simulink model "crane_izka"  (R2021a)
settings: Solver=VariableStepAuto  StartTime=0.0  StopTime=sim_time  FixedStep=sim_step  MaxStep=sim_step  RelTol=1e-3
values from neighbouring files (symbols this model uses):
  C = Pop(i,4)    [GA.m]    (also in izka.mat = 4.74862786183; meranie1.mat = 11.3345130893; meranie2.mat = 10.8395112259; meranie3.mat = 10.5647928076)
  F_cart_den = [0.09763	1	0]    [GA.m]    (also in izka.mat = [2.81374905355e-05 1 0]; meranie1.mat = [2.81374905355e-05 1 0]; meranie2.mat = [2.81374905355e-05 1 0]; meranie3.mat = [2.81374905355e-05 1 0])
  F_cart_num = [0	0	0.3345]    [GA.m]    (also in izka.mat = [0 0 0.21759813997]; meranie1.mat = [0 0 0.21759813997]; meranie2.mat = [0 0 0.21759813997]; meranie3.mat = [0 0 0.21759813997])
  F_pend_den = [1	0.01135	12.54]    [GA.m]    (also in izka.mat = [1 0.0125366535497 12.956800497]; meranie1.mat = [1 0.0125366535497 12.956800497]; meranie2.mat = [1 0.0125366535497 12.956800497]; meranie3.mat = [1 0.0125366535497 12.956800497])
  F_pend_num = [-1.214 0	0]    [GA.m]    (also in izka.mat = [-1.37069413494 0 0]; meranie1.mat = [-1.37069413494 0 0]; meranie2.mat = [-1.37069413494 0 0]; meranie3.mat = [-1.37069413494 0 0])
  I = Pop(i,2)    [GA.m]    (also in izka.mat = 7.78140484293; meranie1.mat = 0.526099986265; meranie2.mat = 3.05318784953; meranie3.mat = 0.594304323923)
  I1 = Pop(i,3)    [GA.m]    (also in meranie_6_4.mat = -16.7252340033)
  l = 0.58    [GA.m]    (also in izka.mat; meranie1.mat; meranie2.mat; meranie3.mat)
  P = Pop(i,1)    [GA.m]    (also in izka.mat = 9.77813174253; meranie1.mat = 6.16880734651; meranie2.mat = 6.25392782724; meranie3.mat = 8.1585790558)
  P1 = 6.16880734651    [meranie1.mat]    (also in meranie2.mat = 6.25392782724)
  sim_step = 0.01    [GA.m]    (also in meranie1.mat; meranie2.mat; meranie3.mat; meranie4-2.mat)
libraries: pid_lib x4, simulink x4, SignalEditorBlockLib x2
settings Model: Creator=maros-pc  LastModifiedBy=maros-pc
settings SolverCC: ConsecutiveZCsStepRelTol=10000*128*eps
settings DebuggingCC: UnconnectedInputMsg=none  UnconnectedOutputMsg=none  UnconnectedLineMsg=none
settings ModelReferenceCC: EnableRefExpFcnMdlSchedulingChecks=off
settings RTWCC: Description=Generic Real-Time Target  DLArmComputeVersion=20.02.1

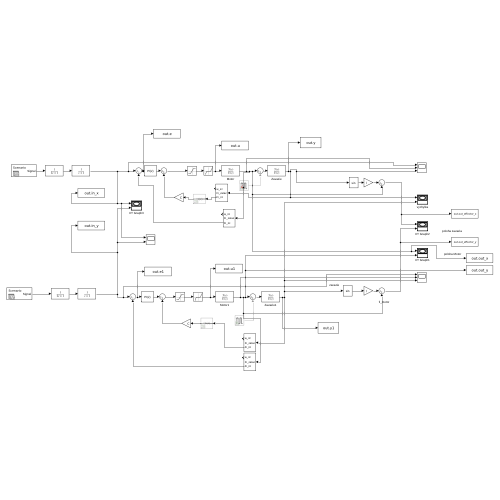
[thumbnail: Simulink's stored preview of the top-level diagram]
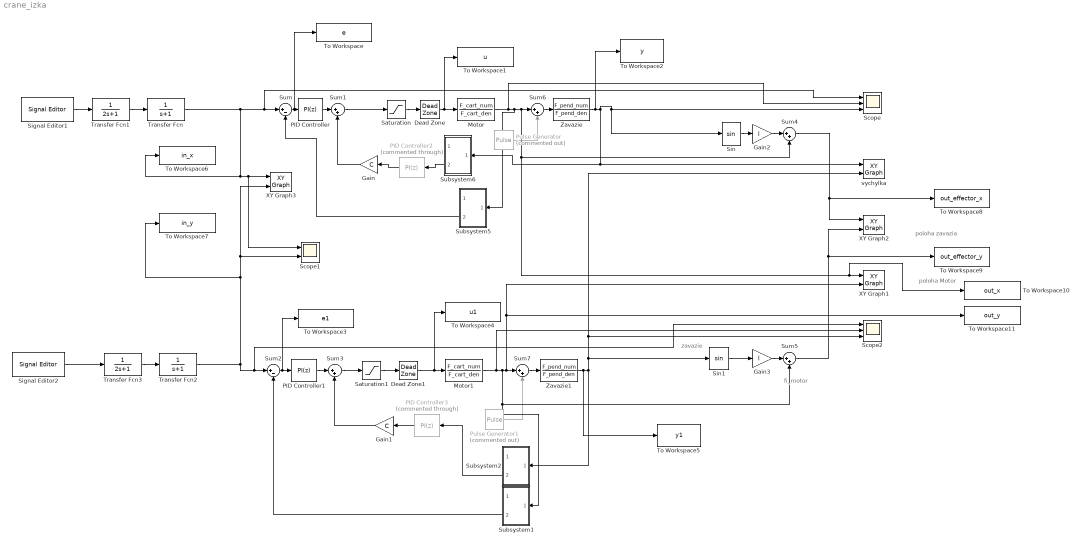
== system crane_izka ==
  note: poloha zavazia
  note: poloha Motor
  note: fi_motor
  note: zavazie
  Dead Zone : DeadZone  LowerValue=-0.2  UpperValue=0.2  SaturateOnIntegerOverflow=on
  Dead Zone1 : DeadZone  LowerValue=-0.2  UpperValue=0.2  SaturateOnIntegerOverflow=on
  Gain : Gain  Gain=C
  Gain1 : Gain  Gain=C
  Gain2 : Gain  Gain=l
  Gain3 : Gain  Gain=l
  Motor : TransferFcn  Numerator=F_cart_num  Denominator=F_cart_den
  Motor1 : TransferFcn  Numerator=F_cart_num  Denominator=F_cart_den
  PID Controller : pid_lib/PID Controller  Controller=PI  Form=Parallel  TimeDomain=Discrete-time  UseExternalTs=off  SampleTime=-1  IntegratorMethod=Forward Euler  FilterMethod=Forward Euler  ControllerParametersSource=internal  P=P  I=I  D=0  N=100  UseFilter=on  TunerSelectOption=Transfer Function Based (PID Tuner App)  InitialConditionSource=internal  InitialConditionForIntegrator=0  InitialConditionForFilter=0  DifferentiatorICPrevScaledInput=0  ExternalReset=none  TrackingMode=off  Kt=1  LimitOutput=off  SatLimitsSource=internal  UpperSaturationLimit=inf  LowerSaturationLimit=-inf  LinearizeAsGain=on  AntiWindupMode=none  Kb=1  POutMin=[]  POutMax=[]  IOutMin=[]  IOutMax=[]  DOutMin=[]  DOutMax=[]  NOutMin=[]  NOutMax=[]  SumOutMin=[]  SumOutMax=[]  SaturationOutMin=[]  SaturationOutMax=[]  PParamMin=[]  PParamMax=[]  IParamMin=[]  IParamMax=[]  DParamMin=[]  DParamMax=[]  NParamMin=[]  NParamMax=[]  KbParamMin=[]  KbParamMax=[]  KtParamMin=[]  KtParamMax=[]  KbOutMin=[]  KbOutMax=[]  KtOutMin=[]  KtOutMax=[]  IntegratorOutMin=[]  IntegratorOutMax=[]  FilterOutMin=[]  FilterOutMax=[]  SumI1OutMin=[]  SumI1OutMax=[]  SumI2OutMin=[]  SumI2OutMax=[]  SumI3OutMin=[]  SumI3OutMax=[]  SumI4OutMin=[]  SumI4OutMax=[]  SumDOutMin=[]  SumDOutMax=[]  DifferentiatorOutMin=[]  DifferentiatorOutMax=[]  FilterDiffOutCoefMin=[]  FilterDiffOutCoefMax=[]  ReciprocalOutMin=[]  ReciprocalOutMax=[]  SumDenOutMin=[]  SumDenOutMax=[]  SumNumOutMin=[]  SumNumOutMax=[]  DivideOutMin=[]  DivideOutMax=[]  UdiffTsProdOutMin=[]  UdiffTsProdOutMax=[]  NTsProdOutMin=[]  NTsProdOutMax=[]  UintegralTsProdOutMin=[]  UintegralTsProdOutMax=[]  UngainTsProdOutMin=[]  UngainTsProdOutMax=[]  IntegratorContinuousStateAttributes=''  IntegratorStateMustResolveToSignalObject=off  IntegratorRTWStateStorageClass=Auto  FilterContinuousStateAttributes=''  FilterStateMustResolveToSignalObject=off  FilterRTWStateStorageClass=Auto  ParallelPVariant=InternalParameters  IdealPVariant=Disabled  IVariant=InternalParameters  DVariant=Disabled  IntegratorVariant=Discrete  SatVariant=Disabled  AWVariant=Passthrough  PCopyVariant=Disabled  TRVariant=Disabled  FdbkBlocksVariant=Forward  IdealPFdbkVariant=Disabled  SatFdbkVariant=Disabled  DerivativeFilterVariant=Disabled  NVariant=Disabled  NCopyVariant=Disabled_SignalSpec  FilterICVariant=Disabled  IntegratorICVariant=InternalICs  ExternalResetVariant=Disabled  TRSumVariant=Passthrough  SumFdbkVariant=Disabled  SumVariant=Sum_PI  TsampFilterVariant=InternalTs  TsampNgainVariant=Passthrough  TsampIntegralVariant=Disabled_SignalSpec  ExternalSaturationOutDataTypeStr=Inherit: Same as second input
  PID Controller1 : pid_lib/PID Controller  Controller=PI  Form=Parallel  TimeDomain=Discrete-time  UseExternalTs=off  SampleTime=-1  IntegratorMethod=Forward Euler  FilterMethod=Forward Euler  ControllerParametersSource=internal  P=P  I=I  D=0  N=100  UseFilter=on  TunerSelectOption=Transfer Function Based (PID Tuner App)  InitialConditionSource=internal  InitialConditionForIntegrator=0  InitialConditionForFilter=0  DifferentiatorICPrevScaledInput=0  ExternalReset=none  TrackingMode=off  Kt=1  LimitOutput=off  SatLimitsSource=internal  UpperSaturationLimit=inf  LowerSaturationLimit=-inf  LinearizeAsGain=on  AntiWindupMode=none  Kb=1  POutMin=[]  POutMax=[]  IOutMin=[]  IOutMax=[]  DOutMin=[]  DOutMax=[]  NOutMin=[]  NOutMax=[]  SumOutMin=[]  SumOutMax=[]  SaturationOutMin=[]  SaturationOutMax=[]  PParamMin=[]  PParamMax=[]  IParamMin=[]  IParamMax=[]  DParamMin=[]  DParamMax=[]  NParamMin=[]  NParamMax=[]  KbParamMin=[]  KbParamMax=[]  KtParamMin=[]  KtParamMax=[]  KbOutMin=[]  KbOutMax=[]  KtOutMin=[]  KtOutMax=[]  IntegratorOutMin=[]  IntegratorOutMax=[]  FilterOutMin=[]  FilterOutMax=[]  SumI1OutMin=[]  SumI1OutMax=[]  SumI2OutMin=[]  SumI2OutMax=[]  SumI3OutMin=[]  SumI3OutMax=[]  SumI4OutMin=[]  SumI4OutMax=[]  SumDOutMin=[]  SumDOutMax=[]  DifferentiatorOutMin=[]  DifferentiatorOutMax=[]  FilterDiffOutCoefMin=[]  FilterDiffOutCoefMax=[]  ReciprocalOutMin=[]  ReciprocalOutMax=[]  SumDenOutMin=[]  SumDenOutMax=[]  SumNumOutMin=[]  SumNumOutMax=[]  DivideOutMin=[]  DivideOutMax=[]  UdiffTsProdOutMin=[]  UdiffTsProdOutMax=[]  NTsProdOutMin=[]  NTsProdOutMax=[]  UintegralTsProdOutMin=[]  UintegralTsProdOutMax=[]  UngainTsProdOutMin=[]  UngainTsProdOutMax=[]  IntegratorContinuousStateAttributes=''  IntegratorStateMustResolveToSignalObject=off  IntegratorRTWStateStorageClass=Auto  FilterContinuousStateAttributes=''  FilterStateMustResolveToSignalObject=off  FilterRTWStateStorageClass=Auto  ParallelPVariant=InternalParameters  IdealPVariant=Disabled  IVariant=InternalParameters  DVariant=Disabled  IntegratorVariant=Discrete  SatVariant=Disabled  AWVariant=Passthrough  PCopyVariant=Disabled  TRVariant=Disabled  FdbkBlocksVariant=Forward  IdealPFdbkVariant=Disabled  SatFdbkVariant=Disabled  DerivativeFilterVariant=Disabled  NVariant=Disabled  NCopyVariant=Disabled_SignalSpec  FilterICVariant=Disabled  IntegratorICVariant=InternalICs  ExternalResetVariant=Disabled  TRSumVariant=Passthrough  SumFdbkVariant=Disabled  SumVariant=Sum_PI  TsampFilterVariant=InternalTs  TsampNgainVariant=Passthrough  TsampIntegralVariant=Disabled_SignalSpec  ExternalSaturationOutDataTypeStr=Inherit: Same as second input
  PID Controller2 : pid_lib/PID Controller  Commented=through  Controller=PI  Form=Parallel  TimeDomain=Discrete-time  UseExternalTs=off  SampleTime=-1  IntegratorMethod=Forward Euler  FilterMethod=Forward Euler  ControllerParametersSource=internal  P=P1  I=I1  D=0  N=100  UseFilter=on  TunerSelectOption=Transfer Function Based (PID Tuner App)  InitialConditionSource=internal  InitialConditionForIntegrator=0  InitialConditionForFilter=0  DifferentiatorICPrevScaledInput=0  ExternalReset=none  TrackingMode=off  Kt=1  LimitOutput=off  SatLimitsSource=internal  UpperSaturationLimit=inf  LowerSaturationLimit=-inf  LinearizeAsGain=on  AntiWindupMode=none  Kb=1  POutMin=[]  POutMax=[]  IOutMin=[]  IOutMax=[]  DOutMin=[]  DOutMax=[]  NOutMin=[]  NOutMax=[]  SumOutMin=[]  SumOutMax=[]  SaturationOutMin=[]  SaturationOutMax=[]  PParamMin=[]  PParamMax=[]  IParamMin=[]  IParamMax=[]  DParamMin=[]  DParamMax=[]  NParamMin=[]  NParamMax=[]  KbParamMin=[]  KbParamMax=[]  KtParamMin=[]  KtParamMax=[]  KbOutMin=[]  KbOutMax=[]  KtOutMin=[]  KtOutMax=[]  IntegratorOutMin=[]  IntegratorOutMax=[]  FilterOutMin=[]  FilterOutMax=[]  SumI1OutMin=[]  SumI1OutMax=[]  SumI2OutMin=[]  SumI2OutMax=[]  SumI3OutMin=[]  SumI3OutMax=[]  SumI4OutMin=[]  SumI4OutMax=[]  SumDOutMin=[]  SumDOutMax=[]  DifferentiatorOutMin=[]  DifferentiatorOutMax=[]  FilterDiffOutCoefMin=[]  FilterDiffOutCoefMax=[]  ReciprocalOutMin=[]  ReciprocalOutMax=[]  SumDenOutMin=[]  SumDenOutMax=[]  SumNumOutMin=[]  SumNumOutMax=[]  DivideOutMin=[]  DivideOutMax=[]  UdiffTsProdOutMin=[]  UdiffTsProdOutMax=[]  NTsProdOutMin=[]  NTsProdOutMax=[]  UintegralTsProdOutMin=[]  UintegralTsProdOutMax=[]  UngainTsProdOutMin=[]  UngainTsProdOutMax=[]  IntegratorContinuousStateAttributes=''  IntegratorStateMustResolveToSignalObject=off  IntegratorRTWStateStorageClass=Auto  FilterContinuousStateAttributes=''  FilterStateMustResolveToSignalObject=off  FilterRTWStateStorageClass=Auto  ParallelPVariant=InternalParameters  IdealPVariant=Disabled  IVariant=InternalParameters  DVariant=Disabled  IntegratorVariant=Discrete  SatVariant=Disabled  AWVariant=Passthrough  PCopyVariant=Disabled  TRVariant=Disabled  FdbkBlocksVariant=Forward  IdealPFdbkVariant=Disabled  SatFdbkVariant=Disabled  DerivativeFilterVariant=Disabled  NVariant=Disabled  NCopyVariant=Disabled_SignalSpec  FilterICVariant=Disabled  IntegratorICVariant=InternalICs  ExternalResetVariant=Disabled  TRSumVariant=Passthrough  SumFdbkVariant=Disabled  SumVariant=Sum_PI  TsampFilterVariant=InternalTs  TsampNgainVariant=Passthrough  TsampIntegralVariant=Disabled_SignalSpec  ExternalSaturationOutDataTypeStr=Inherit: Same as second input
  PID Controller3 : pid_lib/PID Controller  Commented=through  Controller=PI  Form=Parallel  TimeDomain=Discrete-time  UseExternalTs=off  SampleTime=-1  IntegratorMethod=Forward Euler  FilterMethod=Forward Euler  ControllerParametersSource=internal  P=P1  I=I1  D=0  N=100  UseFilter=on  TunerSelectOption=Transfer Function Based (PID Tuner App)  InitialConditionSource=internal  InitialConditionForIntegrator=0  InitialConditionForFilter=0  DifferentiatorICPrevScaledInput=0  ExternalReset=none  TrackingMode=off  Kt=1  LimitOutput=off  SatLimitsSource=internal  UpperSaturationLimit=inf  LowerSaturationLimit=-inf  LinearizeAsGain=on  AntiWindupMode=none  Kb=1  POutMin=[]  POutMax=[]  IOutMin=[]  IOutMax=[]  DOutMin=[]  DOutMax=[]  NOutMin=[]  NOutMax=[]  SumOutMin=[]  SumOutMax=[]  SaturationOutMin=[]  SaturationOutMax=[]  PParamMin=[]  PParamMax=[]  IParamMin=[]  IParamMax=[]  DParamMin=[]  DParamMax=[]  NParamMin=[]  NParamMax=[]  KbParamMin=[]  KbParamMax=[]  KtParamMin=[]  KtParamMax=[]  KbOutMin=[]  KbOutMax=[]  KtOutMin=[]  KtOutMax=[]  IntegratorOutMin=[]  IntegratorOutMax=[]  FilterOutMin=[]  FilterOutMax=[]  SumI1OutMin=[]  SumI1OutMax=[]  SumI2OutMin=[]  SumI2OutMax=[]  SumI3OutMin=[]  SumI3OutMax=[]  SumI4OutMin=[]  SumI4OutMax=[]  SumDOutMin=[]  SumDOutMax=[]  DifferentiatorOutMin=[]  DifferentiatorOutMax=[]  FilterDiffOutCoefMin=[]  FilterDiffOutCoefMax=[]  ReciprocalOutMin=[]  ReciprocalOutMax=[]  SumDenOutMin=[]  SumDenOutMax=[]  SumNumOutMin=[]  SumNumOutMax=[]  DivideOutMin=[]  DivideOutMax=[]  UdiffTsProdOutMin=[]  UdiffTsProdOutMax=[]  NTsProdOutMin=[]  NTsProdOutMax=[]  UintegralTsProdOutMin=[]  UintegralTsProdOutMax=[]  UngainTsProdOutMin=[]  UngainTsProdOutMax=[]  IntegratorContinuousStateAttributes=''  IntegratorStateMustResolveToSignalObject=off  IntegratorRTWStateStorageClass=Auto  FilterContinuousStateAttributes=''  FilterStateMustResolveToSignalObject=off  FilterRTWStateStorageClass=Auto  ParallelPVariant=InternalParameters  IdealPVariant=Disabled  IVariant=InternalParameters  DVariant=Disabled  IntegratorVariant=Discrete  SatVariant=Disabled  AWVariant=Passthrough  PCopyVariant=Disabled  TRVariant=Disabled  FdbkBlocksVariant=Forward  IdealPFdbkVariant=Disabled  SatFdbkVariant=Disabled  DerivativeFilterVariant=Disabled  NVariant=Disabled  NCopyVariant=Disabled_SignalSpec  FilterICVariant=Disabled  IntegratorICVariant=InternalICs  ExternalResetVariant=Disabled  TRSumVariant=Passthrough  SumFdbkVariant=Disabled  SumVariant=Sum_PI  TsampFilterVariant=InternalTs  TsampNgainVariant=Passthrough  TsampIntegralVariant=Disabled_SignalSpec  ExternalSaturationOutDataTypeStr=Inherit: Same as second input
  Pulse Generator : DiscretePulseGenerator  Commented=on  PulseType=Time based  Amplitude=0.1  Period=5
  Pulse Generator1 : DiscretePulseGenerator  Commented=on  PulseType=Time based  Amplitude=0.1  Period=5
  Saturation : Saturate  UpperLimit=1  LowerLimit=-1
  Saturation1 : Saturate  UpperLimit=1  LowerLimit=-1
  Scope : Scope  NumInputPorts=3
  Scope1 : Scope  NumInputPorts=2
  Scope2 : Scope  NumInputPorts=3
  Signal Editor1 : SignalEditorBlockLib/Signal Editor  FileName=ziadana_polohax.mat  ActiveScenario=Scenario  ActiveSignal=Signal  IsBus=off  OutputBusObjectStr=Bus: BusObject  SampleTime=sim_step  Interpolate=off  ZeroCross=off  OutputAfterFinalValue=Holding final value  Unit=inherit  PreserveSignalName=on
  Signal Editor2 : SignalEditorBlockLib/Signal Editor  FileName=ziadana_poloha_y.mat  ActiveScenario=Scenario  ActiveSignal=Signal  IsBus=off  OutputBusObjectStr=Bus: BusObject  SampleTime=0  Interpolate=off  ZeroCross=off  OutputAfterFinalValue=Holding final value  Unit=inherit  PreserveSignalName=on
  Sin : Trigonometry
  Sin1 : Trigonometry
  Subsystem1 : Subsystem
  Subsystem2 : Subsystem
  Subsystem5 : Subsystem
  Subsystem6 : Subsystem
  Sum : Sum  Inputs=|+-
  Sum{1,3..7} (6 alike) : Sum  Inputs=|++
  Sum2 : Sum  Inputs=|+-
  To Workspace : ToWorkspace  VariableName=e  SaveFormat=Timeseries  SampleTime=-1
  To Workspace1 : ToWorkspace  VariableName=u  SaveFormat=Timeseries  SampleTime=-1
  To Workspace10 : ToWorkspace  VariableName=out_x  SaveFormat=Timeseries  SampleTime=-1
  To Workspace11 : ToWorkspace  VariableName=out_y  SaveFormat=Timeseries  SampleTime=-1
  To Workspace2 : ToWorkspace  VariableName=y  SaveFormat=Timeseries  SampleTime=-1
  To Workspace3 : ToWorkspace  VariableName=e1  SaveFormat=Timeseries  SampleTime=-1
  To Workspace4 : ToWorkspace  VariableName=u1  SaveFormat=Timeseries  SampleTime=-1
  To Workspace5 : ToWorkspace  VariableName=y1  SaveFormat=Timeseries  SampleTime=-1
  To Workspace6 : ToWorkspace  VariableName=in_x  SaveFormat=Timeseries  SampleTime=-1
  To Workspace7 : ToWorkspace  VariableName=in_y  SaveFormat=Timeseries  SampleTime=-1
  To Workspace8 : ToWorkspace  VariableName=out_effector_x  SaveFormat=Timeseries  SampleTime=-1
  To Workspace9 : ToWorkspace  VariableName=out_effector_y  SaveFormat=Timeseries  SampleTime=-1
  Transfer Fcn : TransferFcn  Denominator=[1 1]
  Transfer Fcn1 : TransferFcn  Denominator=[2 1]
  Transfer Fcn2 : TransferFcn  Denominator=[1 1]
  Transfer Fcn3 : TransferFcn  Denominator=[2 1]
  XY Graph1 : simulink/Sinks/XY Graph  xmin=-1  xmax=1  ymin=-1  ymax=1  st=-1
  XY Graph2 : simulink/Sinks/XY Graph  xmin=-1  xmax=1  ymin=-1  ymax=1  st=-1
  XY Graph3 : simulink/Sinks/XY Graph  xmin=-1  xmax=1  ymin=-1  ymax=1  st=-1
  Zavazie : TransferFcn  Numerator=F_pend_num  Denominator=F_pend_den
  Zavazie1 : TransferFcn  Numerator=F_pend_num  Denominator=F_pend_den
  vychylka : simulink/Sinks/XY Graph  xmin=-1  xmax=1  ymin=-1  ymax=1  st=-1
  wires:
  Zavazie/1 -> To Workspace2/1, Subsystem6/1(Fi_zataz), vychylka/1, Sin/1, Scope/3
  Motor/1 -> Scope/2, Subsystem5/1(Fi_zataz), Sum4/2, To Workspace10/1, XY Graph1/1, Sum6/1
  Sum/1 -> To Workspace/1, PID Controller/1
  Gain/1 -> Sum1/2
  Saturation/1 -> Dead Zone/1
  Dead Zone/1 -> To Workspace1/1, Motor/1
  PID Controller/1 -> Sum1/1
  Transfer Fcn/1 -> Scope1/1, XY Graph3/1, To Workspace6/1, Scope/1, Sum/1
  Saturation1/1 -> Dead Zone1/1
  Gain1/1 -> Sum3/2
  Dead Zone1/1 -> To Workspace4/1, Motor1/1
  Zavazie1/1 -> To Workspace5/1, Sin1/1, vychylka/2, Scope2/3, Subsystem2/1(Fi_zataz)
  Sum3/1 -> Saturation1/1
  Sum2/1 -> To Workspace3/1, PID Controller1/1
  PID Controller1/1 -> Sum3/1
  Transfer Fcn2/1 -> Scope2/1, Sum2/1, To Workspace7/1, Scope1/2, XY Graph3/2
  Sum4/1 -> To Workspace8/1, XY Graph2/1
  Sum5/1 -> To Workspace9/1, XY Graph2/2
  Sum6/1 -> Zavazie/1
  Pulse Generator/1 -> Sum6/2
  Sin/1 -> Gain2/1
  Gain2/1 -> Sum4/1
  Sin1/1 -> Gain3/1
  Gain3/1 -> Sum5/1
  Subsystem5/2(Fi_irc) -> Sum/2
  Subsystem1/2(Fi_irc) -> Sum2/2
  Transfer Fcn1/1 -> Transfer Fcn/1
  Signal Editor1/1 -> Transfer Fcn1/1
  Transfer Fcn3/1 -> Transfer Fcn2/1
  Signal Editor2/1 -> Transfer Fcn3/1
  Sum1/1 -> Saturation/1
  Sum7/1 -> Zavazie1/1
  Pulse Generator1/1 -> Sum7/2
  PID Controller2/1 -> Gain/1
  PID Controller3/1 -> Gain1/1
  Subsystem2/2(Fi_irc) -> PID Controller3/1
  Subsystem6/2(Fi_irc) -> PID Controller2/1
  Motor1/1 -> Scope2/2, Sum7/1, XY Graph1/2, To Workspace11/1, Sum5/2, Subsystem1/1(Fi_zataz)

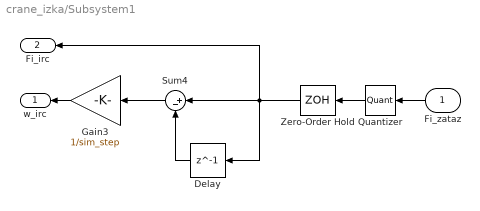
== system crane_izka/Subsystem1 ==
  Fi_zataz : Inport
  Delay : Delay  DelayLength=1
  Gain3 : Gain  Gain=1/sim_step
  Quantizer : Quantizer  QuantizationInterval=5.8157e-5
  Sum4 : Sum  Inputs=|+-
  Zero-Order Hold : ZeroOrderHold  SampleTime=sim_step
  w_irc : Outport
  Fi_irc : Outport  Port=2
  wires:
  Sum4/1 -> Gain3/1
  Delay/1 -> Sum4/2
  Zero-Order Hold/1 -> Delay/1, Sum4/1, Fi_irc/1
  Fi_zataz/1 -> Quantizer/1
  Quantizer/1 -> Zero-Order Hold/1
  Gain3/1 -> w_irc/1

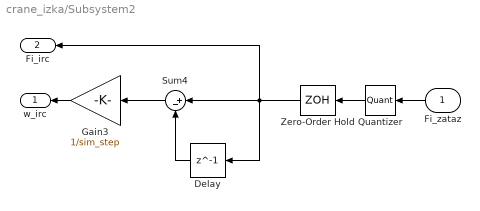
== system crane_izka/Subsystem2 ==
  Fi_zataz : Inport
  Delay : Delay  DelayLength=1
  Gain3 : Gain  Gain=1/sim_step
  Quantizer : Quantizer  QuantizationInterval=15e-4
  Sum4 : Sum  Inputs=|+-
  Zero-Order Hold : ZeroOrderHold  SampleTime=sim_step
  w_irc : Outport
  Fi_irc : Outport  Port=2
  wires:
  Sum4/1 -> Gain3/1
  Delay/1 -> Sum4/2
  Zero-Order Hold/1 -> Delay/1, Sum4/1, Fi_irc/1
  Fi_zataz/1 -> Quantizer/1
  Quantizer/1 -> Zero-Order Hold/1
  Gain3/1 -> w_irc/1

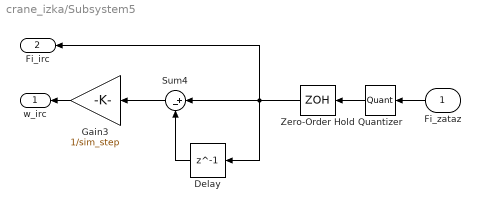
== system crane_izka/Subsystem5 ==
  Fi_zataz : Inport
  Delay : Delay  DelayLength=1
  Gain3 : Gain  Gain=1/sim_step
  Quantizer : Quantizer  QuantizationInterval=5.8157e-5
  Sum4 : Sum  Inputs=|+-
  Zero-Order Hold : ZeroOrderHold  SampleTime=sim_step
  w_irc : Outport
  Fi_irc : Outport  Port=2
  wires:
  Sum4/1 -> Gain3/1
  Delay/1 -> Sum4/2
  Zero-Order Hold/1 -> Delay/1, Sum4/1, Fi_irc/1
  Fi_zataz/1 -> Quantizer/1
  Quantizer/1 -> Zero-Order Hold/1
  Gain3/1 -> w_irc/1

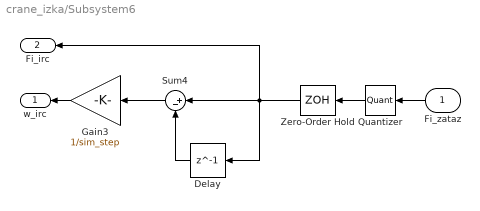
== system crane_izka/Subsystem6 ==
  Fi_zataz : Inport
  Delay : Delay  DelayLength=1
  Gain3 : Gain  Gain=1/sim_step
  Quantizer : Quantizer  QuantizationInterval=15e-4
  Sum4 : Sum  Inputs=|+-
  Zero-Order Hold : ZeroOrderHold  SampleTime=sim_step
  w_irc : Outport
  Fi_irc : Outport  Port=2
  wires:
  Sum4/1 -> Gain3/1
  Delay/1 -> Sum4/2
  Zero-Order Hold/1 -> Delay/1, Sum4/1, Fi_irc/1
  Fi_zataz/1 -> Quantizer/1
  Quantizer/1 -> Zero-Order Hold/1
  Gain3/1 -> w_irc/1
